simulink model "slide26"  (R2021a)
settings: Solver=VariableStepAuto  StartTime=0.0  StopTime=10.0  RelTol=1e-3
settings Model: Creator=MarcosRPesanteColón  LastModifiedBy=MarcosRPesanteColón

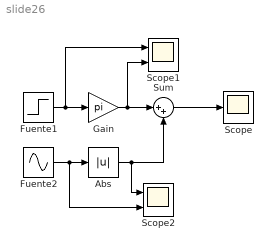
== system slide26 ==
  Abs : Abs
  Fuente1 : Step  SampleTime=0
  Fuente2 : Sin  Frequency=pi  SampleTime=0
  Gain : Gain  Gain=pi
  Scope : Scope
  Scope1 : Scope  NumInputPorts=2
  Scope2 : Scope  NumInputPorts=2
  Sum : Sum  Inputs=|++
  wires:
  Sum/1 -> Scope/1
  Fuente2/1 -> Scope2/2, Abs/1
  Abs/1 -> Scope2/1, Sum/2
  Fuente1/1 -> Scope1/1, Gain/1
  Gain/1 -> Scope1/2, Sum/1
